simulink model "cs_proj_cl_ramp"  (R2021b)
settings: Solver=ode4  StartTime=0.0  StopTime=10.0  FixedStep=0.001  RelTol=1e-3
values from neighbouring files (symbols this model uses):
  K = 5    [cs_project_2.m]    (also in cs_project_3.m; cs_project_5.m; cs_project_6.m; cs_project_7.m)
libraries: simulink x1
settings Model: Creator=shash  LastModifiedBy=shash
settings DataIOCC: ReturnWorkspaceOutputs=off

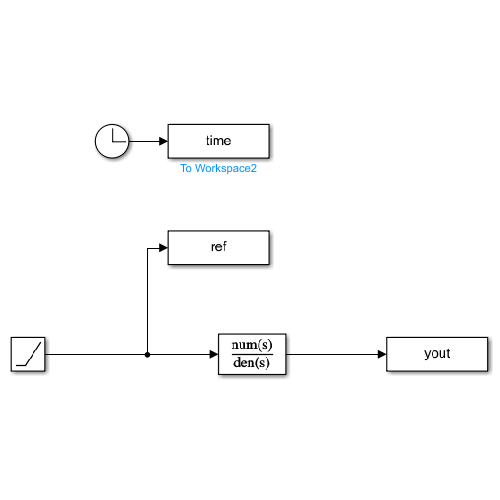
[thumbnail: Simulink's stored preview of the top-level diagram]
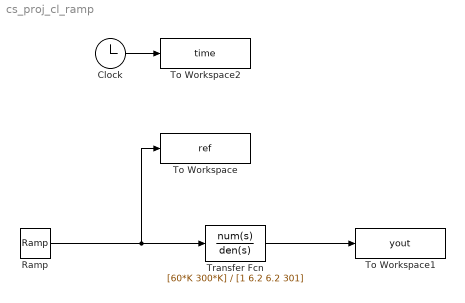
== system cs_proj_cl_ramp ==
  Clock : Clock
  Ramp : simulink/Sources/Ramp  slope=1  start=0  InitialOutput=0
  To Workspace : ToWorkspace  VariableName=ref  SampleTime=-1
  To Workspace1 : ToWorkspace  VariableName=yout  SampleTime=-1
  To Workspace2 : ToWorkspace  VariableName=time  SampleTime=-1
  Transfer Fcn : TransferFcn  Numerator=[60*K 300*K]  Denominator=[1 6.2 6.2 301]
  wires:
  Transfer Fcn/1 -> To Workspace1/1
  Ramp/1 -> To Workspace/1, Transfer Fcn/1
  Clock/1 -> To Workspace2/1
